simulink model "newController"  (R2023a)
settings: Solver=VariableStepAuto  StartTime=0.0  StopTime=10.0  RelTol=1e-3
libraries: ros2lib x65
(part 1 of 2)
settings Model: Creator=john  LastModifiedBy=john

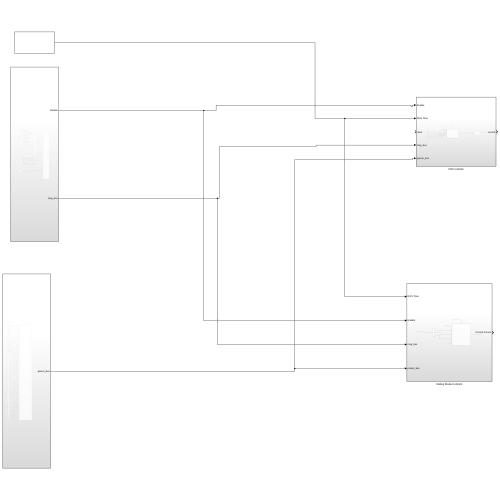
[thumbnail: Simulink's stored preview of the top-level diagram]
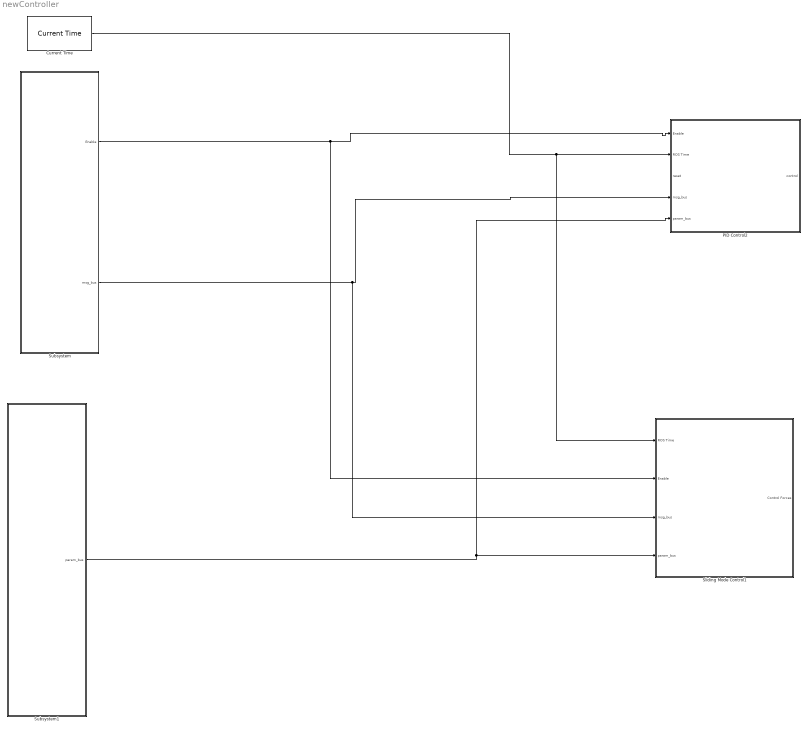
== system newController ==
  Current Time : ros2lib/Current Time  OutputFormat=bus  SampleTime=-1  ModelName=untitled
  PID Control2 : Subsystem
  Sliding Mode Control1 : Subsystem
  Subsystem : Subsystem
  Subsystem1 : Subsystem
  wires:
  Subsystem/2(msg_bus) -> Sliding Mode Control1/3(msg_bus), PID Control2/4(msg_bus)
  Subsystem1/1(param_bus) -> Sliding Mode Control1/4(param_bus), PID Control2/5(param_bus)
  Subsystem/1(Enable) -> Sliding Mode Control1/2(Enable), PID Control2/1(Enable)
  Current Time/1 -> Sliding Mode Control1/1(ROS Time), PID Control2/2(ROS Time)

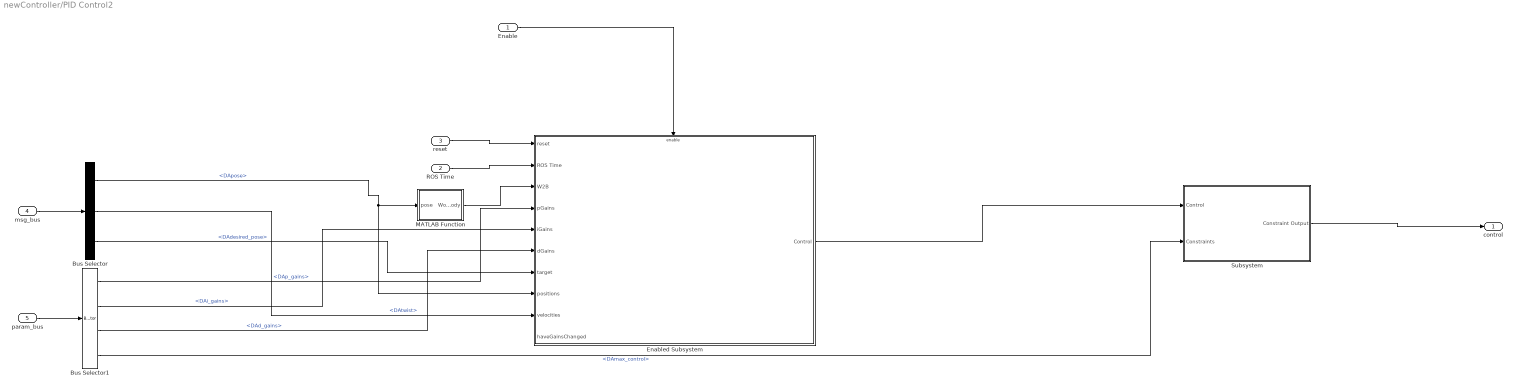
== system newController/PID Control2 ==
  Enable : Inport
  ROS Time : Inport  Port=2
  reset : Inport  Port=3
  msg_bus : Inport  Port=4
  param_bus : Inport  Port=5
  Bus Selector : BusSelector  OutputSignals=current_state.DApose,current_state.DAtwist,desired_pose.DAdesired_pose
  Bus Selector1 : BusSelector  OutputSignals=DAp_gains,DAi_gains,DAd_gains,DAmax_control
  Enabled Subsystem : Subsystem  TreatAsAtomicUnit=on
  MATLAB Function : MATLAB Function  TreatAsAtomicUnit=on
  Subsystem : Subsystem
  control : Outport
  wires:
  param_bus/1 -> Bus Selector1/1
  Enable/1 -> Enabled Subsystem/Enable
  reset/1 -> Enabled Subsystem/1(reset)
  ROS Time/1 -> Enabled Subsystem/2(ROS Time)
  Bus Selector1/1 -> Enabled Subsystem/4(pGains)  "<DAp_gains>"
  Bus Selector1/2 -> Enabled Subsystem/5(iGains)  "<DAi_gains>"
  Bus Selector1/3 -> Enabled Subsystem/6(dGains)  "<DAd_gains>"
  Bus Selector1/4 -> Subsystem/2(Constraints)  "<DAmax_control>"
  msg_bus/1 -> Bus Selector/1
  Bus Selector/1 -> MATLAB Function/1(pose), Enabled Subsystem/8(positions)  "<DApose>"
  Bus Selector/2 -> Enabled Subsystem/9(velocities)  "<DAtwist>"
  Bus Selector/3 -> Enabled Subsystem/7(target)  "<DAdesired_pose>"
  MATLAB Function/1(World2Body) -> Enabled Subsystem/3(W2B)
  Subsystem/1(Constraint Output) -> control/1
  Enabled Subsystem/1(Control) -> Subsystem/1(Control)

== system newController/Sliding Mode Control1 ==
  ROS Time : Inport
  Enable : Inport  Port=2
  msg_bus : Inport  Port=3
  param_bus : Inport  Port=4
  Bus Selector : BusSelector  OutputSignals=current_state.DApose,current_state.DAtwist,desired_pose.DAdesired_pose
  Subsystem : Subsystem
  Control Forces : Outport
  wires:
  msg_bus/1 -> Bus Selector/1
  ROS Time/1 -> Subsystem/1(ROS Time)
  Enable/1 -> Subsystem/Enable
  Bus Selector/1 -> Subsystem/2(Current Positions)  "<DApose>"
  Bus Selector/2 -> Subsystem/3(World Velocities)  "<DAtwist>"
  Bus Selector/3 -> Subsystem/4(Target Positions)  "<DAdesired_pose>"
  param_bus/1 -> Subsystem/5(param_bus)
  Subsystem/1(Control Forces) -> Control Forces/1

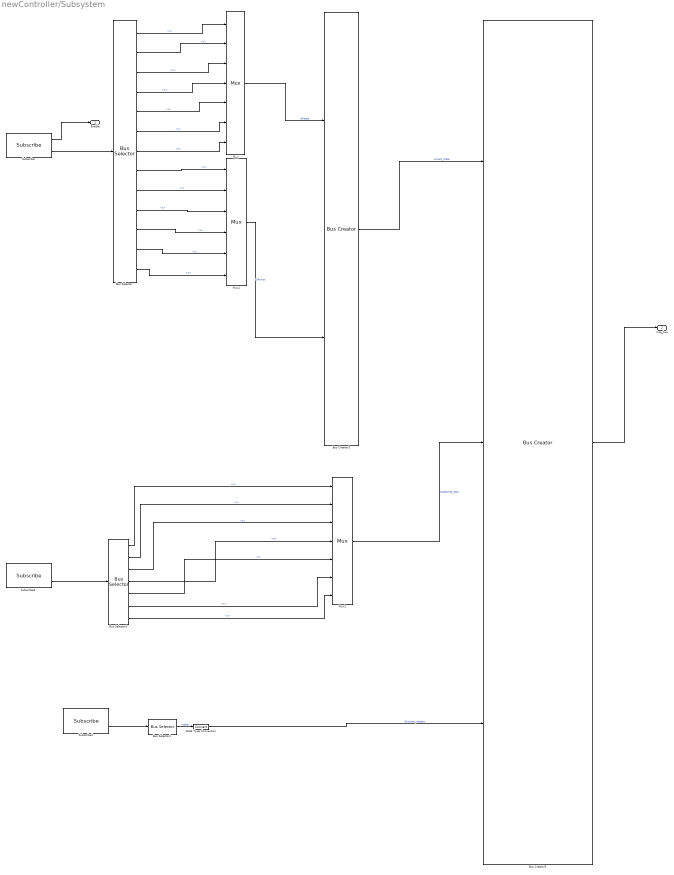
== system newController/Subsystem ==
  Bus Creator3 : BusCreator  Inputs=2
  Bus Creator5 : BusCreator  Inputs=3
  Bus Selector : BusSelector  OutputSignals=pose.pose.position.x,pose.pose.position.y,pose.pose.position.z,pose.pose.orientation.w,pose.pose.orientation.x,pose.pose.orientation.y,pose.pose.orientation.z,twist.twist.linear.x,twist.twist.linear.y,twist.twist.linear.z,twist.twist.angular.x,twist.twist.angular.y,twist.twist.angular.z
  Bus Selector1 : BusSelector  OutputSignals=data
  Bus Selector2 : BusSelector  OutputSignals=setpoint_vect.x,setpoint_vect.y,setpoint_vect.z,setpoint_quat.w,setpoint_quat.x,setpoint_quat.y,setpoint_quat.z
  Data Type Conversion : DataTypeConversion  SaturateOnIntegerOverflow=off  RndMeth=Floor
  Mux : Mux  Inputs=7
  Mux1 : Mux  Inputs=6
  Mux2 : Mux  Inputs=7
  Subscribe : ros2lib/Subscribe  topicSource=Specify your own  topic=/mercury/odometry/filtered  messageType=nav_msgs/Odometry  sampleTime=-1  QOSHistory=Keep last  QOSDepth=1  QOSReliability=Reliable  QOSDurability=Volatile
  Subscribe1 : ros2lib/Subscribe  topicSource=Specify your own  topic=/talos/controller/solver_weights  messageType=std_msgs/Int32MultiArray  sampleTime=-1  QOSHistory=Keep last  QOSDepth=1  QOSReliability=Reliable  QOSDurability=Volatile
      settings: LibrarySourceBlock=roslib/ROS 2/Subscribe
  Subscribe4 : ros2lib/Subscribe  topicSource=Specify your own  topic=/mercury/controller/desired  messageType=riptide_msgs2/ControllerCommand  sampleTime=-1  QOSHistory=Keep last  QOSDepth=1  QOSReliability=Reliable  QOSDurability=Volatile
  Enable : Outport
  msg_bus : Outport  Port=2
  wires:
  Subscribe/1 -> Enable/1
  Subscribe/2 -> Bus Selector/1
  Bus Selector/2 -> Mux/2  "<y>"
  Bus Selector/1 -> Mux/1  "<x>"
  Bus Selector/3 -> Mux/3  "<z>"
  Bus Selector/4 -> Mux/4  "<w>"
  Bus Selector/5 -> Mux/5  "<x>"
  Bus Selector/6 -> Mux/6  "<y>"
  Bus Selector/7 -> Mux/7  "<z>"
  Mux/1 -> Bus Creator3/1  "DApose"
  Bus Selector/8 -> Mux1/1  "<x>"
  Bus Selector/9 -> Mux1/2  "<y>"
  Bus Selector/10 -> Mux1/3  "<z>"
  Bus Selector/11 -> Mux1/4  "<x>"
  Bus Selector/12 -> Mux1/5  "<y>"
  Bus Selector/13 -> Mux1/6  "<z>"
  Mux1/1 -> Bus Creator3/2  "DAtwist"
  Subscribe4/2 -> Bus Selector2/1
  Bus Selector2/1 -> Mux2/1  "<x>"
  Bus Selector2/2 -> Mux2/2  "<y>"
  Bus Selector2/3 -> Mux2/3  "<z>"
  Bus Selector2/4 -> Mux2/4  "<w>"
  Bus Selector2/5 -> Mux2/5  "<x>"
  Bus Selector2/6 -> Mux2/6  "<y>"
  Bus Selector2/7 -> Mux2/7  "<z>"
  Bus Creator3/1 -> Bus Creator5/1  "current_state"
  Mux2/1 -> Bus Creator5/2  "DAdesired_pose"
  Bus Creator5/1 -> msg_bus/1
  Data Type Conversion/1 -> Bus Creator5/3  "DAsolver_weights"
  Subscribe1/2 -> Bus Selector1/1
  Bus Selector1/1 -> Data Type Conversion/1  "<data>"

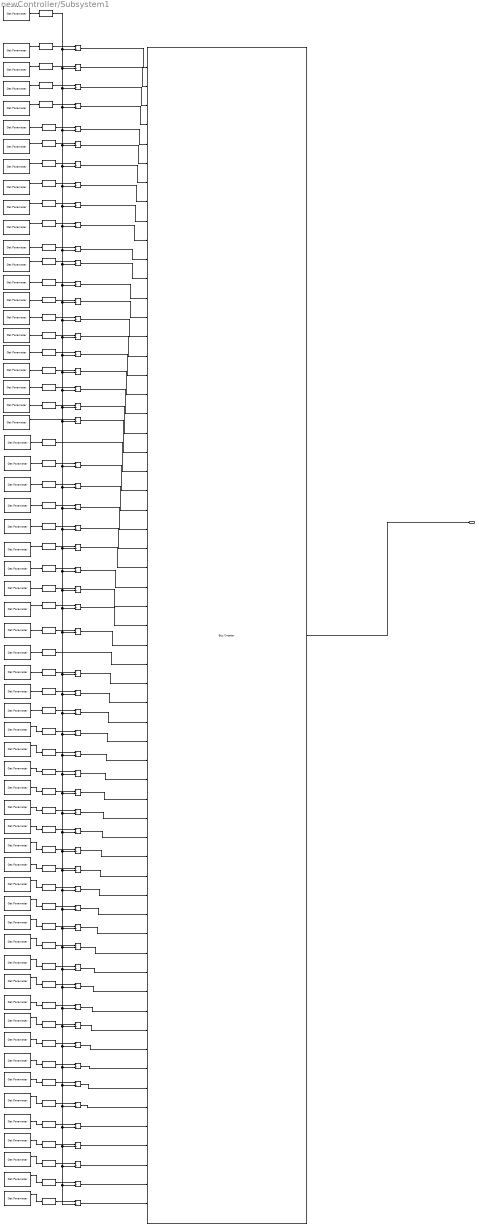
== system newController/Subsystem1 ==
  Active Input Mask : ros2lib/Get Parameter  ParameterName=controller__active_force_mask  ParameterType=int64[]  ParameterMaxArrayLength=6  ParameterInitialValue=[0,0,0,0,0,0]  SampleTime=-1  ModelName=mercury  BlockId=ParamGet_mercury_181
  Bsnt_safe_mode : DataTypeConversion  OutDataTypeStr=boolean  SaturateOnIntegerOverflow=off  RndMeth=Floor
  Bts_table_mode : DataTypeConversion  OutDataTypeStr=boolean  SaturateOnIntegerOverflow=off  RndMeth=Floor
  DAauto_tune_initial : Product  Inputs=*/
  DAauto_tune_mask : Product  Inputs=*/
  DAd_gains : Product  Inputs=*/
  DAi_gains : Product  Inputs=*/
  DAmax_control : Product  Inputs=*/
  DAnominal_variance : Product  Inputs=*/
  DAp_gains : Product  Inputs=*/
  DAsmc_eta_0 : Product  Inputs=*/
  DAsmc_eta_1 : Product  Inputs=*/
  DAsmc_lamda : Product  Inputs=*/
  DAsmc_max_accelerations : Product  Inputs=*/
  DAsmc_velocity_curve : Product  Inputs=*/
  DAtele_nudge_forces : Product  Inputs=*/
  DAts_rpm_coefficients : Product  Inputs=*/
  DAts_wrenchmat : Product  Inputs=*/
  Data Type Conversion{1,4..14,16..18,20..23} (19 alike) : DataTypeConversion  OutDataTypeStr=double  SaturateOnIntegerOverflow=off  RndMeth=Floor
  Dnominal_time{,1..17} (18 alike) : Product  Inputs=*/
  Dpositional_error_threshold : Product  Inputs=*/
  Dreset_threshold : Product  Inputs=*/
  Dreset_trust_threshold : Product  Inputs=*/
  Dreset_weight_minimum : Product  Inputs=*/
  Dsnt_barrel_roll_duration : Product  Inputs=*/
  Dsnt_barrel_roll_force : Product  Inputs=*/
  Dsnt_summersault_duration : Product  Inputs=*/
  Dsnt_summersault_force : Product  Inputs=*/
  Dtele_accel_force : Product  Inputs=*/
  Dtele_boost_cooldown : Product  Inputs=*/
  Dtele_boost_duration : Product  Inputs=*/
  Dtele_boost_multiplier : Product  Inputs=*/
  Dtele_drag_coefficient : Product  Inputs=*/
  Dtele_reverse_multiplier : Product  Inputs=*/
  Dtele_steering_angle : Product  Inputs=*/
  Dtele_throttle_deadzone : Product  Inputs=*/
  Dtele_width : Product  Inputs=*/
  Dtrust_decay_tau : Product  Inputs=*/
  Dtrust_growth_tau : Product  Inputs=*/
  Dts_disable_weight : Product  Inputs=*/
  Dts_feedback_decay : Product  Inputs=*/
  Dts_individual_thrust_limit : Product  Inputs=*/
  Dts_thrust_limit : Product  Inputs=*/
  Dvelocity_threshold : Product  Inputs=*/
  Eta 0 : ros2lib/Get Parameter  ParameterName=controller__SMC__SMC_params__eta_order_0  ParameterType=int64[]  ParameterMaxArrayLength=6  ParameterInitialValue=0.0  SampleTime=-1  ModelName=mercury  BlockId=ParamGet_mercury_260
      settings: LibrarySourceBlock=roslib/ROS 2/Get Parameter
  Eta 1 : ros2lib/Get Parameter  ParameterName=controller__SMC__SMC_params__eta_order_1  ParameterType=int64[]  ParameterMaxArrayLength=6  ParameterInitialValue=0.0  SampleTime=-1  ModelName=mercury  BlockId=ParamGet_mercury_261
      settings: LibrarySourceBlock=roslib/ROS 2/Get Parameter
  Force To Double{,1..38} (39 alike) : DataTypeConversion  OutDataTypeStr=double  SaturateOnIntegerOverflow=off  RndMeth=Floor
  Force To RPM Curve Parameters : ros2lib/Get Parameter  ParameterName=thruster_solver__force_to_rpm_coefficents  ParameterType=int64[]  ParameterMaxArrayLength=8  ParameterInitialValue=[0,0,0,0,0,0,0,0]  SampleTime=-1  ModelName=mercury  BlockId=ParamGet_mercury_301
      settings: LibrarySourceBlock=roslib/ROS 2/Get Parameter
  Get Parameter10 : ros2lib/Get Parameter  ParameterName=controller__pid__reset_threshold  ParameterType=int64  ParameterMaxArrayLength=16  ParameterInitialValue=100000  SampleTime=-1  ModelName=mercury  BlockId=ParamGet_mercury_302
      settings: LibrarySourceBlock=roslib/ROS 2/Get Parameter
  Get Parameter11 : ros2lib/Get Parameter  ParameterName=controller__teleop__width  ParameterType=int64  ParameterMaxArrayLength=16  ParameterInitialValue=900000  SampleTime=-1  ModelName=mercury  BlockId=ParamGet_mercury_303
  Get Parameter13 : ros2lib/Get Parameter  ParameterName=controller__stunt__summersault_duration  ParameterType=int64  ParameterMaxArrayLength=16  ParameterInitialValue=5000000.0  SampleTime=-1  ModelName=mercury  BlockId=ParamGet_mercury_304
  Get Parameter14 : ros2lib/Get Parameter  ParameterName=controller__stunt__summersault_force  ParameterType=int64  ParameterMaxArrayLength=16  ParameterInitialValue=20000000  SampleTime=-1  ModelName=mercury  BlockId=ParamGet_mercury_305
  Get Parameter15 : ros2lib/Get Parameter  ParameterName=controller__stunt__barrel_roll_duration  ParameterType=int64  ParameterMaxArrayLength=16  ParameterInitialValue=4000000.0  SampleTime=-1  ModelName=mercury  BlockId=ParamGet_mercury_306
  Get Parameter16 : ros2lib/Get Parameter  ParameterName=controller__teleop__boost__cooldown  ParameterType=int64  ParameterMaxArrayLength=16  ParameterInitialValue=10000000  SampleTime=-1  ModelName=mercury  BlockId=ParamGet_mercury_307
  Get Parameter17 : ros2lib/Get Parameter  ParameterName=controller__teleop__boost__duration  ParameterType=int64  ParameterMaxArrayLength=16  ParameterInitialValue=5000000  SampleTime=-1  ModelName=mercury  BlockId=ParamGet_mercury_308
  Get Parameter18 : ros2lib/Get Parameter  ParameterName=controller__teleop__boost__multiplier  ParameterType=int64  ParameterMaxArrayLength=16  ParameterInitialValue=1500000  SampleTime=-1  ModelName=mercury  BlockId=ParamGet_mercury_309
  Get Parameter19 : ros2lib/Get Parameter  ParameterName=controller__teleop__max_steering_angle  ParameterType=int64  ParameterMaxArrayLength=16  ParameterInitialValue=45000000  SampleTime=-1  ModelName=mercury  BlockId=ParamGet_mercury_310
  Get Parameter20 : ros2lib/Get Parameter  ParameterName=controller__teleop__nudge_forces  ParameterType=int64[]  ParameterMaxArrayLength=6  ParameterInitialValue=[20000000, 20000000, 2000000, 200000, 200000, 2000000]  SampleTime=-1  ModelName=mercury  BlockId=ParamGet_mercury_311
  Get Parameter21 : ros2lib/Get Parameter  ParameterName=controller__teleop__throttle_deadzone  ParameterType=int64  ParameterMaxArrayLength=16  ParameterInitialValue=50000  SampleTime=-1  ModelName=mercury  BlockId=ParamGet_mercury_312
  Get Parameter22 : ros2lib/Get Parameter  ParameterName=controller__teleop__reverse_force_multiplier  ParameterType=int64  ParameterMaxArrayLength=16  ParameterInitialValue=400000  SampleTime=-1  ModelName=mercury  BlockId=ParamGet_mercury_313
  Get Parameter23 : ros2lib/Get Parameter  ParameterName=controller__teleop__drag_coefficient  ParameterType=int64  ParameterMaxArrayLength=16  ParameterInitialValue=420000000  SampleTime=-1  ModelName=mercury  BlockId=ParamGet_mercury_314
  Get Parameter24 : ros2lib/Get Parameter  ParameterName=controller__teleop__accel_force  ParameterType=int64  ParameterMaxArrayLength=16  ParameterInitialValue=20000000  SampleTime=-1  ModelName=mercury  BlockId=ParamGet_mercury_315
  Get Parameter25 : ros2lib/Get Parameter  ParameterName=controller__stunt__safe_mode  ParameterType=boolean  ParameterMaxArrayLength=16  ParameterInitialValue=0  SampleTime=-1  ModelName=mercury  BlockId=ParamGet_mercury_316
  Get Parameter26 : ros2lib/Get Parameter  ParameterName=controller__stunt__barrel_roll_force  ParameterType=int64  ParameterMaxArrayLength=16  ParameterInitialValue=25000000.0  SampleTime=-1  ModelName=mercury  BlockId=ParamGet_mercury_317
  Get Thruster Wrench Matrix : ros2lib/Get Parameter  ParameterName=talos_wrenchmat  ParameterType=int64[]  ParameterMaxArrayLength=48  ParameterInitialValue=0.0  SampleTime=-1  ModelName=mercury  BlockId=ParamGet_mercury_318
      settings: LibrarySourceBlock=roslib/ROS 2/Get Parameter
  Iactive_input_mask : Product  Inputs=*/
  Individual Limit : ros2lib/Get Parameter  ParameterName=thruster_solver__individual_thrust_limit  ParameterType=int64  ParameterMaxArrayLength=16  ParameterInitialValue=5.0  SampleTime=-1  ModelName=mercury  BlockId=ParamGet_mercury_320
      settings: LibrarySourceBlock=roslib/ROS 2/Get Parameter
  Individual Limit1 : ros2lib/Get Parameter  ParameterName=thruster_solver__disable_weight  ParameterType=int64  ParameterMaxArrayLength=16  ParameterInitialValue=10000000  SampleTime=-1  ModelName=mercury  BlockId=ParamGet_mercury_321
      settings: LibrarySourceBlock=roslib/ROS 2/Get Parameter
  Individual Limit2 : ros2lib/Get Parameter  ParameterName=thruster_solver_table_mode  ParameterType=boolean  ParameterMaxArrayLength=16  ParameterInitialValue=false  SampleTime=-1  ModelName=mercury  BlockId=ParamGet_mercury_322
      settings: LibrarySourceBlock=roslib/ROS 2/Get Parameter
  Individual Limit3 : ros2lib/Get Parameter  ParameterName=thruster_solver__feedback_decay  ParameterType=int64  ParameterMaxArrayLength=16  ParameterInitialValue=1250000  SampleTime=-1  ModelName=mercury  BlockId=ParamGet_mercury_323
      settings: LibrarySourceBlock=roslib/ROS 2/Get Parameter
  Param Bus : BusCreator  Inputs=60
  Scaling Factor : ros2lib/Get Parameter  ParameterName=controller__SMC__SMC_params__scaling_factor  ParameterType=int64  ParameterMaxArrayLength=16  ParameterInitialValue=1000000  SampleTime=-1  ModelName=mercury  BlockId=ParamGet_mercury_325
      settings: LibrarySourceBlock=roslib/ROS 2/Get Parameter
  System Limit : ros2lib/Get Parameter  ParameterName=thruster_solver__system_thrust_limit  ParameterType=int64  ParameterMaxArrayLength=16  ParameterInitialValue=10  SampleTime=-1  ModelName=mercury  BlockId=ParamGet_mercury_326
      settings: LibrarySourceBlock=roslib/ROS 2/Get Parameter
  convergence threshold1 : ros2lib/Get Parameter  ParameterName=controller__feed_forward__auto_tune__auto_tune_mask  ParameterType=int64[]  ParameterMaxArrayLength=6  ParameterInitialValue=[0;0;0;0;0;0]  SampleTime=-1  ModelName=mercury  BlockId=ParamGet_mercury_327
      settings: LibrarySourceBlock=roslib/ROS 2/Get Parameter
  convergence threshold10 : ros2lib/Get Parameter  ParameterName=controller__feed_forward__auto_tune__trust_threshold  ParameterType=int64[]  ParameterMaxArrayLength=6  ParameterInitialValue=[970000, 970000, 970000, 970000, 970000, 970000]  SampleTime=-1  ModelName=mercury  BlockId=ParamGet_mercury_328
      settings: LibrarySourceBlock=roslib/ROS 2/Get Parameter
  convergence threshold11 : ros2lib/Get Parameter  ParameterName=controller__feed_forward__auto_tune__variation_threshold  ParameterType=int64[]  ParameterMaxArrayLength=6  ParameterInitialValue=[1000000, 1000000, 1000000, 1000000, 1000000, 1000000]  SampleTime=-1  ModelName=mercury  BlockId=ParamGet_mercury_329
      settings: LibrarySourceBlock=roslib/ROS 2/Get Parameter
  convergence threshold12 : ros2lib/Get Parameter  ParameterName=controller__feed_forward__auto_tune__axis_weights  ParameterType=int64[]  ParameterMaxArrayLength=6  ParameterInitialValue=[1000000, 1000000, 1000000, 1000000, 1000000, 1000000]  SampleTime=-1  ModelName=mercury  BlockId=ParamGet_mercury_330
      settings: LibrarySourceBlock=roslib/ROS 2/Get Parameter
  convergence threshold13 : ros2lib/Get Parameter  ParameterName=controller__feed_forward__auto_tune__variation_der_threshold  ParameterType=int64[]  ParameterMaxArrayLength=6  ParameterInitialValue=[1000000, 1000000, 1000000, 1000000, 1000000, 1000000]  SampleTime=-1  ModelName=mercury  BlockId=ParamGet_mercury_331
      settings: LibrarySourceBlock=roslib/ROS 2/Get Parameter
  convergence threshold14 : ros2lib/Get Parameter  ParameterName=inertia  ParameterType=int64[]  ParameterMaxArrayLength=3  ParameterInitialValue=[700000,1590000,1650000]  SampleTime=-1  ModelName=mercury  BlockId=ParamGet_mercury_332
      settings: LibrarySourceBlock=roslib/ROS 2/Get Parameter
  convergence threshold15 : ros2lib/Get Parameter  ParameterName=mass  ParameterType=int64  ParameterMaxArrayLength=6  ParameterInitialValue=32000000  SampleTime=-1  ModelName=mercury  BlockId=ParamGet_mercury_333
      settings: LibrarySourceBlock=roslib/ROS 2/Get Parameter
  convergence threshold16 : ros2lib/Get Parameter  ParameterName=controller__drag_compensator__apply_mask  ParameterType=int64[]  ParameterMaxArrayLength=36  ParameterInitialValue=zeros(36,1)  SampleTime=-1  ModelName=mercury  BlockId=ParamGet_mercury_334
      settings: LibrarySourceBlock=roslib/ROS 2/Get Parameter
  convergence threshold17 : ros2lib/Get Parameter  ParameterName=controller__drag_compensator__minimum_samples  ParameterType=int64  ParameterMaxArrayLength=6  ParameterInitialValue=60000000  SampleTime=-1  ModelName=mercury  BlockId=ParamGet_mercury_335
      settings: LibrarySourceBlock=roslib/ROS 2/Get Parameter
  convergence threshold18 : ros2lib/Get Parameter  ParameterName=controller__drag_compensator__minimum_absolute_velocity  ParameterType=int64  ParameterMaxArrayLength=6  ParameterInitialValue=200000  SampleTime=-1  ModelName=mercury  BlockId=ParamGet_mercury_336
      settings: LibrarySourceBlock=roslib/ROS 2/Get Parameter
  convergence threshold19 : ros2lib/Get Parameter  ParameterName=controller__drag_compensator__minimum_absolute_positional_error  ParameterType=int64  ParameterMaxArrayLength=3  ParameterInitialValue=200000  SampleTime=-1  ModelName=mercury  BlockId=ParamGet_mercury_337
      settings: LibrarySourceBlock=roslib/ROS 2/Get Parameter
  convergence threshold2 : ros2lib/Get Parameter  ParameterName=auto_ff__auto_ff  ParameterType=int64[]  ParameterMaxArrayLength=6  ParameterInitialValue=[0;0;0;0;0;0]  SampleTime=-1  ModelName=mercury  BlockId=ParamGet_mercury_338
      settings: LibrarySourceBlock=roslib/ROS 2/Get Parameter
  convergence threshold20 : ros2lib/Get Parameter  ParameterName=controller__drag_compensator__minimum_average_sampled_velocity  ParameterType=int64[]  ParameterMaxArrayLength=6  ParameterInitialValue=[100000,100000,100000,100000,100000,100000]  SampleTime=-1  ModelName=mercury  BlockId=ParamGet_mercury_339
      settings: LibrarySourceBlock=roslib/ROS 2/Get Parameter
  convergence threshold21 : ros2lib/Get Parameter  ParameterName=controller__drag_compensator__minimum_R2_coeffiecent  ParameterType=int64  ParameterMaxArrayLength=6  ParameterInitialValue=700000  SampleTime=-1  ModelName=mercury  BlockId=ParamGet_mercury_340
      settings: LibrarySourceBlock=roslib/ROS 2/Get Parameter
  convergence threshold22 : ros2lib/Get Parameter  ParameterName=controller__drag_compensator__learning_rate  ParameterType=int64  ParameterMaxArrayLength=6  ParameterInitialValue=200000  SampleTime=-1  ModelName=mercury  BlockId=ParamGet_mercury_341
      settings: LibrarySourceBlock=roslib/ROS 2/Get Parameter
  convergence threshold23 : ros2lib/Get Parameter  ParameterName=controller__drag_compensator__initial_compensation__forward  ParameterType=int64[]  ParameterMaxArrayLength=36  ParameterInitialValue=zeros(36,1)  SampleTime=-1  ModelName=mercury  BlockId=ParamGet_mercury_342
      settings: LibrarySourceBlock=roslib/ROS 2/Get Parameter
  convergence threshold24 : ros2lib/Get Parameter  ParameterName=controller__autoff__initial_ff  ParameterType=int64[]  ParameterMaxArrayLength=6  ParameterInitialValue=[0,0,0,0,0,0,0]  SampleTime=-1  ModelName=mercury  BlockId=ParamGet_mercury_343
      settings: LibrarySourceBlock=roslib/ROS 2/Get Parameter
  convergence threshold25 : ros2lib/Get Parameter  ParameterName=controller__drag_compensator__initial_compensation__reverse  ParameterType=int64[]  ParameterMaxArrayLength=36  ParameterInitialValue=zeros(36,1)  SampleTime=-1  ModelName=mercury  BlockId=ParamGet_mercury_344
      settings: LibrarySourceBlock=roslib/ROS 2/Get Parameter
  convergence threshold3 : ros2lib/Get Parameter  ParameterName=controller__controller_scale__trust_decay_tau  ParameterType=int64  ParameterMaxArrayLength=6  ParameterInitialValue=1000000  SampleTime=-1  ModelName=mercury  BlockId=ParamGet_mercury_345
      settings: LibrarySourceBlock=roslib/ROS 2/Get Parameter
  convergence threshold4 : ros2lib/Get Parameter  ParameterName=controller__controller_scale__trust_growth_tau  ParameterType=int64  ParameterMaxArrayLength=6  ParameterInitialValue=1000000  SampleTime=-1  ModelName=mercury  BlockId=ParamGet_mercury_346
      settings: LibrarySourceBlock=roslib/ROS 2/Get Parameter
  convergence threshold5 : ros2lib/Get Parameter  ParameterName=controller__controller_scale__reset_trust_threshold  ParameterType=int64  ParameterMaxArrayLength=200000  ParameterInitialValue=200000  SampleTime=-1  ModelName=mercury  BlockId=ParamGet_mercury_347
      settings: LibrarySourceBlock=roslib/ROS 2/Get Parameter
  convergence threshold6 : ros2lib/Get Parameter  ParameterName=controller__controller_scale__reset_weight_minimum  ParameterType=int64  ParameterMaxArrayLength=6  ParameterInitialValue=3000000  SampleTime=-1  ModelName=mercury  BlockId=ParamGet_mercury_348
      settings: LibrarySourceBlock=roslib/ROS 2/Get Parameter
  convergence threshold7 : ros2lib/Get Parameter  ParameterName=controller__controller_scale__nominal_variance  ParameterType=int64[]  ParameterMaxArrayLength=6  ParameterInitialValue=[0;0;0;0;0;0]  SampleTime=-1  ModelName=mercury  BlockId=ParamGet_mercury_349
      settings: LibrarySourceBlock=roslib/ROS 2/Get Parameter
  convergence threshold8 : ros2lib/Get Parameter  ParameterName=controller__controller_scale__nominal_time  ParameterType=int64  ParameterMaxArrayLength=6  ParameterInitialValue=3000000  SampleTime=-1  ModelName=mercury  BlockId=ParamGet_mercury_350
      settings: LibrarySourceBlock=roslib/ROS 2/Get Parameter
  convergence threshold9 : ros2lib/Get Parameter  ParameterName=controller__feed_forward__auto_tune__decay_factor  ParameterType=int64[]  ParameterMaxArrayLength=6  ParameterInitialValue=[200000, 200000, 200000, 200000, 200000, 200000]  SampleTime=-1  ModelName=mercury  BlockId=ParamGet_mercury_351
      settings: LibrarySourceBlock=roslib/ROS 2/Get Parameter
  d Gains : ros2lib/Get Parameter  ParameterName=controller__PID__d_gains  ParameterType=int64[]  ParameterMaxArrayLength=6  ParameterInitialValue=[0,0,0,0,0,0]  SampleTime=-1  ModelName=mercury  BlockId=ParamGet_mercury_352
      settings: LibrarySourceBlock=roslib/ROS 2/Get Parameter
  error threshold : ros2lib/Get Parameter  ParameterName=controller__feed_forward__auto_tune__positional_error_threshold  ParameterType=int64  ParameterMaxArrayLength=16  ParameterInitialValue=100000  SampleTime=-1  ModelName=mercury  BlockId=ParamGet_mercury_353
      settings: LibrarySourceBlock=roslib/ROS 2/Get Parameter
  i Gains : ros2lib/Get Parameter  ParameterName=controller__PID__i_gains  ParameterType=int64[]  ParameterMaxArrayLength=6  ParameterInitialValue=[0,0,0,0,0,0]  SampleTime=-1  ModelName=mercury  BlockId=ParamGet_mercury_354
      settings: LibrarySourceBlock=roslib/ROS 2/Get Parameter
  mass1 : ros2lib/Get Parameter  ParameterName=controller__SMC__SMC_params__velocity_curve_params  ParameterType=int64[]  ParameterMaxArrayLength=12  ParameterInitialValue=[0,0,0,0,0,0,0,0,0,0,0,0]  SampleTime=-1  ModelName=mercury  BlockId=ParamGet_mercury_355
      settings: LibrarySourceBlock=roslib/ROS 2/Get Parameter
  mass2 : ros2lib/Get Parameter  ParameterName=controller__SMC__max_target_accelerations  ParameterType=int64[]  ParameterMaxArrayLength=6  ParameterInitialValue=[10000,10000,10000,10000,10000,10000]  SampleTime=-1  ModelName=mercury  BlockId=ParamGet_mercury_356
      settings: LibrarySourceBlock=roslib/ROS 2/Get Parameter
  mass5 : ros2lib/Get Parameter  ParameterName=controller__SMC__SMC_params__lambda  ParameterType=int64[]  ParameterMaxArrayLength=6  ParameterInitialValue=0.0  SampleTime=-1  ModelName=mercury  BlockId=ParamGet_mercury_357
      settings: LibrarySourceBlock=roslib/ROS 2/Get Parameter
  max_control : ros2lib/Get Parameter  ParameterName=controller__PID__max_control_thresholds  ParameterType=int64[]  ParameterMaxArrayLength=6  ParameterInitialValue=[0,0,0,0,0,0]  SampleTime=-1  ModelName=mercury  BlockId=ParamGet_mercury_358
      settings: LibrarySourceBlock=roslib/ROS 2/Get Parameter
  p Gains : ros2lib/Get Parameter  ParameterName=controller__PID__p_gains  ParameterType=int64[]  ParameterMaxArrayLength=6  ParameterInitialValue=[0,0,0,0,0,0]  SampleTime=-1  ModelName=mercury  BlockId=ParamGet_mercury_359
      settings: LibrarySourceBlock=roslib/ROS 2/Get Parameter
  velocity threshold : ros2lib/Get Parameter  ParameterName=controller__feed_forward__auto_tune__velocity_threshold  ParameterType=int64  ParameterMaxArrayLength=16  ParameterInitialValue=100000  SampleTime=-1  ModelName=mercury  BlockId=ParamGet_mercury_360
      settings: LibrarySourceBlock=roslib/ROS 2/Get Parameter
  param_bus : Outport
  wires:
  Force To Double33/1 -> Dnominal_time10/1
  Data Type Conversion22/1 -> Dtele_boost_cooldown/1
  Force To Double30/1 -> Dnominal_time4/1
  Dsnt_barrel_roll_force/1 -> Param Bus/25  "Dsnt_barrel_roll_force"
  mass2/1 -> Data Type Conversion23/1
  p Gains/1 -> Force To Double6/1
  convergence threshold22/1 -> Force To Double35/1
  Dnominal_time13/1 -> Param Bus/55  "DAminimum_drag_update_velocity"
  Dnominal_time10/1 -> Param Bus/52  "Iminimum_drag_samples"
  Data Type Conversion7/1 -> DAsmc_eta_1/1
  Dnominal_time7/1 -> Param Bus/50  "Dmass"
  Force To Double26/1 -> Dnominal_time/1
  Eta 1/1 -> Data Type Conversion7/1
  Force To Double37/1 -> Dnominal_time16/1
  Force To Double20/1 -> DAauto_tune_initial/1
  Force To Double34/1 -> Dnominal_time8/1
  convergence threshold24/1 -> Force To Double37/1
  Data Type Conversion17/1 -> Dsnt_summersault_duration/1
  Dsnt_summersault_duration/1 -> Param Bus/24  "Dsnt_summersault_duration"
  convergence threshold17/1 -> Force To Double33/1
  Data Type Conversion16/1 -> Dsnt_summersault_force/1
  Dreset_threshold/1 -> Param Bus/5  "Dreset_threshold"
  Force To Double14/1 -> Dnominal_time5/1
  DAp_gains/1 -> Param Bus/2  "DAp_gains"
  System Limit/1 -> Force To Double1/1
  Dnominal_time2/1 -> Param Bus/45  "DAautoff_measurement_trust_threshold"
  Dnominal_time8/1 -> Param Bus/56  "Ddrag_minimum_correspondence_coeffiecent"
  Force To Double35/1 -> Dnominal_time14/1
  Force To Double9/1 -> Dreset_threshold/1
  Dtele_throttle_deadzone/1 -> Param Bus/11  "Dtele_throttle_deadzone"
  DAsmc_lamda/1 -> Param Bus/6  "DAsmc_lamda"
  convergence threshold23/1 -> Force To Double36/1
  Data Type Conversion5/1 -> DAsmc_lamda/1
  Dnominal_time9/1 -> Param Bus/51  "IAdrag_apply_mask"
  convergence threshold7/1 -> Force To Double25/1
  Data Type Conversion20/1 -> Dtele_boost_multiplier/1
  Dtele_steering_angle/1 -> Param Bus/13  "Dtele_steering_angle"
  Get Parameter22/1 -> Data Type Conversion13/1
  Dnominal_time14/1 -> Param Bus/57  "Ddrag_learning_rate"
  Get Parameter19/1 -> Data Type Conversion9/1
  DAtele_nudge_forces/1 -> Param Bus/12  "DAtele_nudge_forces"
  Dtele_reverse_multiplier/1 -> Param Bus/17  "Dtele_reverse_multiplier"
  Dnominal_time16/1 -> Param Bus/59  "DAautoff_init_compensation"
  Dreset_weight_minimum/1 -> Param Bus/41  "Dreset_weight_minimum"
  Force To Double1/1 -> Dts_thrust_limit/1
  Get Parameter25/1 -> Bsnt_safe_mode/1
  DAsmc_max_accelerations/1 -> Param Bus/10  "DAsmc_max_accelerations"
  Force To Double17/1 -> Dnominal_time11/1
  Data Type Conversion18/1 -> Dsnt_barrel_roll_force/1
  convergence threshold10/1 -> Force To Double28/1
  Get Parameter11/1 -> Data Type Conversion10/1
  convergence threshold16/1 -> Force To Double32/1
  Get Parameter16/1 -> Data Type Conversion22/1
  convergence threshold6/1 -> Force To Double24/1
  convergence threshold3/1 -> Force To Double21/1
  DAts_rpm_coefficients/1 -> Param Bus/30  "DAts_rpm_coefficients"
  Force To Double38/1 -> Dnominal_time17/1
  Dtele_boost_cooldown/1 -> Param Bus/20  "Dtele_boost_cooldown"
  Data Type Conversion6/1 -> DAsmc_eta_0/1
  Force To Double2/1 -> Dts_individual_thrust_limit/1
  Force To Double21/1 -> Dtrust_decay_tau/1
  Data Type Conversion11/1 -> Dtele_accel_force/1
  DAts_wrenchmat/1 -> Param Bus/27  "DAts_wrenchmat"
  convergence threshold2/1 -> Force To Double20/1
  Force To Double5/1 -> Dts_disable_weight/1
  Force To Double3/1 -> Dtele_throttle_deadzone/2, DAtele_nudge_forces/2, Dtele_steering_angle/2, Dtele_width/2, Dtele_accel_force/2, Dtele_drag_coefficient/2, Dtele_boost_multiplier/2, Dtele_boost_duration/2, Dtele_boost_cooldown/2, Dsnt_summersault_force/2, Dsnt_summersault_duration/2, Dsnt_barrel_roll_duration/2, DAts_wrenchmat/2, Dts_thrust_limit/2, Dts_individual_thrust_limit/2, DAts_rpm_coefficients/2, Dvelocity_threshold/2, Dtrust_decay_tau/2, Dtrust_growth_tau/2, Dreset_trust_threshold/2, Dreset_weight_minimum/2, DAnominal_variance/2, Dnominal_time17/2, Dnominal_time16/2, Dnominal_time15/2, Dnominal_time14/2, Dnominal_time8/2, Dnominal_time13/2, Dnominal_time12/2, Dnominal_time11/2, Dnominal_time10/2, Dnominal_time9/2, Dnominal_time7/2, Dnominal_time6/2, Dnominal_time5/2, Dnominal_time4/2, Dnominal_time3/2, Dnominal_time2/2, Dnominal_time1/2, Dnominal_time/2, DAauto_tune_initial/2, DAauto_tune_mask/2, Dpositional_error_threshold/2, Dts_feedback_decay/2, Dts_disable_weight/2, Dsnt_barrel_roll_force/2, Iactive_input_mask/2, Dtele_reverse_multiplier/2, DAsmc_max_accelerations/2, DAsmc_velocity_curve/2, DAsmc_eta_1/2, DAsmc_eta_0/2, DAsmc_lamda/2, Dreset_threshold/2, DAi_gains/2, DAd_gains/2, DAp_gains/2, DAmax_control/2
  Data Type Conversion10/1 -> Dtele_width/1
  DAsmc_velocity_curve/1 -> Param Bus/9  "DAsmc_velocity_curve"
  Force To Double15/1 -> Dnominal_time7/1
  Dnominal_time/1 -> Param Bus/43  "Dnominal_time"
  Get Parameter20/1 -> Data Type Conversion8/1
  convergence threshold1/1 -> Force To Double19/1
  Individual Limit/1 -> Force To Double2/1
  Dtele_drag_coefficient/1 -> Param Bus/16  "Dtele_drag_coefficient"
  Get Parameter21/1 -> Data Type Conversion4/1
  Force To Double22/1 -> Dtrust_growth_tau/1
  Dts_thrust_limit/1 -> Param Bus/28  "Dts_thrust_limit"
  Bsnt_safe_mode/1 -> Param Bus/22  "Bsnt_safe_mode"
  i Gains/1 -> Force To Double8/1
  convergence threshold12/1 -> Force To Double30/1
  Param Bus/1 -> param_bus/1
  Scaling Factor/1 -> Force To Double3/1
  Force To Double10/1 -> Dts_feedback_decay/1
  Data Type Conversion21/1 -> Dtele_boost_duration/1
  Dtele_accel_force/1 -> Param Bus/15  "Dtele_accel_force"
  Data Type Conversion13/1 -> Dtele_reverse_multiplier/1
  Force To Double8/1 -> DAi_gains/1
  Dts_individual_thrust_limit/1 -> Param Bus/29  "Dts_individual_thrust_limit"
  convergence threshold11/1 -> Force To Double29/1
  Data Type Conversion1/1 -> DAsmc_velocity_curve/1
  Get Parameter18/1 -> Data Type Conversion20/1
  convergence threshold21/1 -> Force To Double34/1
  Dnominal_time11/1 -> Param Bus/53  "Dminimum_drag_sampling_velocity"
  convergence threshold9/1 -> Force To Double27/1
  convergence threshold8/1 -> Force To Double26/1
  Dnominal_time15/1 -> Param Bus/58  "DAdrag_init_compensation_forward"
  convergence threshold15/1 -> Force To Double15/1
  Force To RPM Curve Parameters/1 -> Force To Double4/1
  convergence threshold5/1 -> Force To Double23/1
  Dsnt_summersault_force/1 -> Param Bus/23  "Dsnt_summersault_force"
  Force To Double11/1 -> DAmax_control/1
  Get Parameter10/1 -> Force To Double9/1
  mass1/1 -> Data Type Conversion1/1
  Dnominal_time1/1 -> Param Bus/44  "DAautoff_body_force_decay_percentage"
  DAauto_tune_mask/1 -> Param Bus/36  "DAauto_tune_mask"
  Data Type Conversion23/1 -> DAsmc_max_accelerations/1
  max_control/1 -> Force To Double11/1
  Dnominal_time3/1 -> Param Bus/46  "DAautoff_standard_variation_threshold"
  Bts_table_mode/1 -> Param Bus/32  "Bts_table_mode"
  Force To Double29/1 -> Dnominal_time3/1
  Dtele_boost_duration/1 -> Param Bus/19  "Dtele_boost_duration"
  Iactive_input_mask/1 -> Param Bus/21  "Iactive_input_mask"
  Get Thruster Wrench Matrix/1 -> Force To Double/1
  convergence threshold4/1 -> Force To Double22/1
  Data Type Conversion9/1 -> Dtele_steering_angle/1
  Data Type Conversion4/1 -> Dtele_throttle_deadzone/1
  d Gains/1 -> Force To Double7/1
  Force To Double24/1 -> Dreset_weight_minimum/1
  DAsmc_eta_1/1 -> Param Bus/8  "DAsmc_eta_1"
  Force To Double7/1 -> DAd_gains/1
  Individual Limit2/1 -> Bts_table_mode/1
  Data Type Conversion8/1 -> DAtele_nudge_forces/1
  Force To Double23/1 -> Dreset_trust_threshold/1
  Force To Double6/1 -> DAp_gains/1
  Get Parameter13/1 -> Data Type Conversion17/1
  Data Type Conversion12/1 -> Dtele_drag_coefficient/1
  Dnominal_time4/1 -> Param Bus/47  "DAautoff_active_force_weights"
  Dts_disable_weight/1 -> Param Bus/31  "Dts_disable_weight"
  Get Parameter24/1 -> Data Type Conversion11/1
  DAd_gains/1 -> Param Bus/3  "DAd_gains"
  Dtrust_decay_tau/1 -> Param Bus/38  "Dtrust_decay_tau"
  Force To Double4/1 -> DAts_rpm_coefficients/1
  DAmax_control/1 -> Param Bus/1  "DAmax_control"
  Dpositional_error_threshold/1 -> Param Bus/34  "Dpositional_error_threshold"
  Get Parameter14/1 -> Data Type Conversion16/1
  Force To Double16/1 -> Dnominal_time6/1
  Dvelocity_threshold/1 -> Param Bus/35  "Dvelocity_threshold"
  velocity threshold/1 -> Force To Double13/1
  Dtele_boost_multiplier/1 -> Param Bus/18  "Dtele_boost_multiplier"
  convergence threshold18/1 -> Force To Double17/1
  Force To Double12/1 -> Dpositional_error_threshold/1
  Force To Double/1 -> DAts_wrenchmat/1
  Data Type Conversion14/1 -> Dsnt_barrel_roll_duration/1
  DAauto_tune_initial/1 -> Param Bus/37  "DAauto_tune_initial"
  DAsmc_eta_0/1 -> Param Bus/7  "DAsmc_eta_0"
  Dreset_trust_threshold/1 -> Param Bus/40  "Dreset_trust_threshold"
  DAnominal_variance/1 -> Param Bus/42  "DAnominal_variance"
  Dtrust_growth_tau/1 -> Param Bus/39  "Dtrust_growth_tau"
  Dnominal_time12/1 -> Param Bus/54  "Dminimum_drag_positional_error"
  Force To Double27/1 -> Dnominal_time1/1
  Individual Limit3/1 -> Force To Double10/1
  Force To Double19/1 -> DAauto_tune_mask/1
  Force To Double36/1 -> Dnominal_time15/1
  Active Input Mask/1 -> Iactive_input_mask/1
  convergence threshold20/1 -> Force To Double18/1
  mass5/1 -> Data Type Conversion5/1
  Force To Double13/1 -> Dvelocity_threshold/1
  Force To Double31/1 -> Dnominal_time12/1
  Individual Limit1/1 -> Force To Double5/1
  Dts_feedback_decay/1 -> Param Bus/33  "Dts_feedback_decay"
  Dnominal_time5/1 -> Param Bus/48  "DAautoff_variation_derivative_threshold"
  Get Parameter23/1 -> Data Type Conversion12/1
  Eta 0/1 -> Data Type Conversion6/1
  Dtele_width/1 -> Param Bus/14  "Dtele_width"
  convergence threshold14/1 -> Force To Double16/1
  Dnominal_time6/1 -> Param Bus/49  "DAinterias"
  Get Parameter15/1 -> Data Type Conversion14/1
  convergence threshold19/1 -> Force To Double31/1
  DAi_gains/1 -> Param Bus/4  "DAi_gains"
  convergence threshold25/1 -> Force To Double38/1
  Get Parameter17/1 -> Data Type Conversion21/1
  Force To Double18/1 -> Dnominal_time13/1
  Force To Double25/1 -> DAnominal_variance/1
  Force To Double32/1 -> Dnominal_time9/1
  convergence threshold13/1 -> Force To Double14/1
  Dnominal_time17/1 -> Param Bus/60  "DAdrag_init_compensation_reverse"
  error threshold/1 -> Force To Double12/1
  Dsnt_barrel_roll_duration/1 -> Param Bus/26  "Dsnt_barrel_roll_duration"
  Force To Double28/1 -> Dnominal_time2/1
  Get Parameter26/1 -> Data Type Conversion18/1

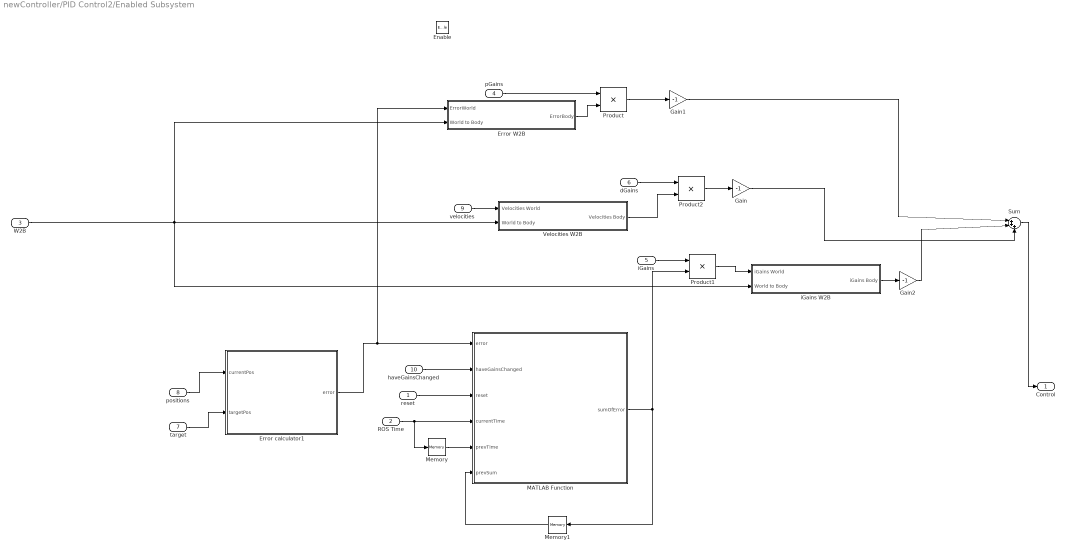
== system newController/PID Control2/Enabled Subsystem ==
  reset : Inport
  ROS Time : Inport  Port=2
  W2B : Inport  Port=3
  pGains : Inport  Port=4
  iGains : Inport  Port=5
  dGains : Inport  Port=6
  target : Inport  Port=7
  positions : Inport  Port=8
  velocities : Inport  Port=9
  haveGainsChanged : Inport  Port=10
  Enable : EnablePort
  Error W2B : Subsystem
  Error calculator1 : MATLAB Function  TreatAsAtomicUnit=on
  Gain : Gain  Gain=-1
  Gain1 : Gain  Gain=-1
  Gain2 : Gain  Gain=-1
  MATLAB Function : MATLAB Function  TreatAsAtomicUnit=on
  Memory : Memory  InheritSampleTime=on
  Memory1 : Memory  InheritSampleTime=on
  Product : Product
  Product1 : Product
  Product2 : Product
  Sum : Sum  Inputs=|+++
  Velocities W2B : Subsystem
  iGains W2B : Subsystem
  Control : Outport
  wires:
  positions/1 -> Error calculator1/1(currentPos)
  target/1 -> Error calculator1/2(targetPos)
  Error calculator1/1(error) -> MATLAB Function/1(error), Error W2B/1(ErrorWorld)
  reset/1 -> MATLAB Function/3(reset)
  ROS Time/1 -> Memory/1, MATLAB Function/4(currentTime)
  haveGainsChanged/1 -> MATLAB Function/2(haveGainsChanged)
  Memory/1 -> MATLAB Function/5(prevTime)
  MATLAB Function/1(sumOfError) -> Product1/2, Memory1/1
  Memory1/1 -> MATLAB Function/6(prevSum)
  iGains/1 -> Product1/1
  velocities/1 -> Velocities W2B/1(Velocities World)
  Product2/1 -> Gain/1
  Product/1 -> Gain1/1
  Gain/1 -> Sum/3
  Sum/1 -> Control/1
  dGains/1 -> Product2/1
  W2B/1 -> iGains W2B/2(World to Body), Velocities W2B/2(World to Body), Error W2B/2(World to Body)
  Error W2B/1(ErrorBody) -> Product/2
  pGains/1 -> Product/1
  iGains W2B/1(iGains Body) -> Gain2/1
  Product1/1 -> iGains W2B/1(iGains World)
  Velocities W2B/1(Velocities Body) -> Product2/2
  Gain1/1 -> Sum/1
  Gain2/1 -> Sum/2

== system newController/PID Control2/Subsystem ==
  Control : Inport
  Constraints : Inport  Port=2
  Gain : Gain  Gain=-1
  MinMax : MinMax  Function=max  Inputs=2
  MinMax1 : MinMax  Inputs=2
  Constraint Output : Outport
  wires:
  Constraints/1 -> MinMax1/2, Gain/1
  Gain/1 -> MinMax/2
  Control/1 -> MinMax/1
  MinMax/1 -> MinMax1/1
  MinMax1/1 -> Constraint Output/1

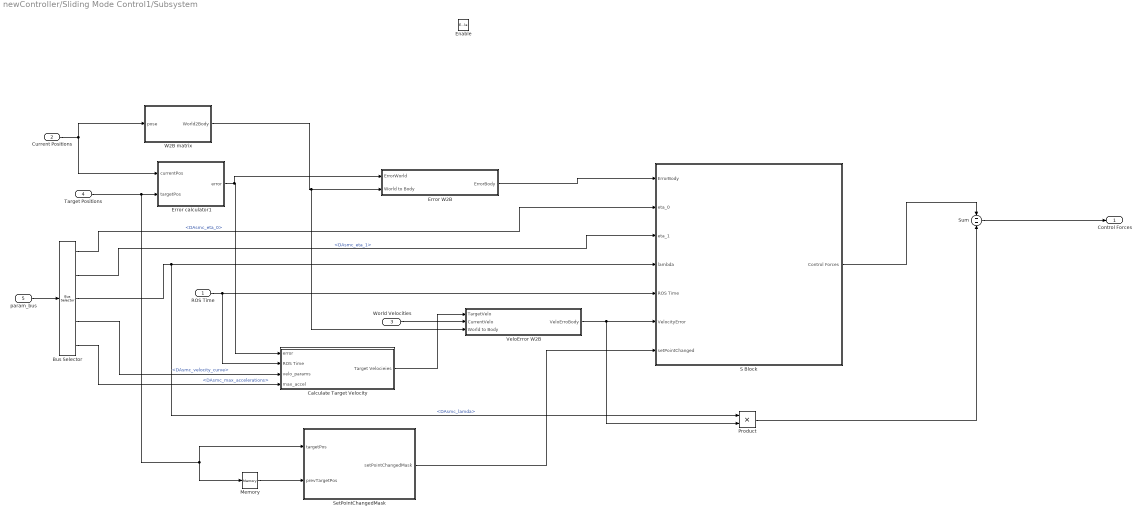
== system newController/Sliding Mode Control1/Subsystem ==
  ROS Time : Inport
  Current Positions : Inport  Port=2
  World Velocities : Inport  Port=3
  Target Positions : Inport  Port=4
  param_bus : Inport  Port=5
  Enable : EnablePort
  Bus Selector : BusSelector  OutputSignals=DAsmc_eta_0,DAsmc_eta_1,DAsmc_lamda,DAsmc_velocity_curve,DAsmc_max_accelerations
  Calculate Target Velocity : Subsystem
  Error W2B : Subsystem
  Error calculator1 : MATLAB Function  TreatAsAtomicUnit=on
  Memory : Memory
  Product : Product
  S Block : Subsystem
  SetPointChangedMask : MATLAB Function  TreatAsAtomicUnit=on
  Sum : Sum  Inputs=--
  VeloError W2B : Subsystem
  W2B matrix : MATLAB Function  TreatAsAtomicUnit=on
  Control Forces : Outport
  wires:
  Target Positions/1 -> Memory/1, SetPointChangedMask/1(targetPos), Error calculator1/2(targetPos)
  Current Positions/1 -> W2B matrix/1(pose), Error calculator1/1(currentPos)
  ROS Time/1 -> Calculate Target Velocity/2(ROS Time), S Block/5(ROS Time)
  Error calculator1/1(error) -> Error W2B/1(ErrorWorld), Calculate Target Velocity/1(error)
  param_bus/1 -> Bus Selector/1
  Bus Selector/5 -> Calculate Target Velocity/4(max_accel)  "<DAsmc_max_accelerations>"
  Bus Selector/4 -> Calculate Target Velocity/3(velo_params)  "<DAsmc_velocity_curve>"
  Bus Selector/2 -> S Block/3(eta_1)  "<DAsmc_eta_1>"
  Bus Selector/1 -> S Block/2(eta_0)  "<DAsmc_eta_0>"
  Bus Selector/3 -> S Block/4(lambda), Product/1  "<DAsmc_lamda>"
  World Velocities/1 -> VeloError W2B/2(CurrentVelo)
  Calculate Target Velocity/1(Target Velocieies) -> VeloError W2B/1(TargetVelo)
  Error W2B/1(ErrorBody) -> S Block/1(ErrorBody)
  W2B matrix/1(World2Body) -> VeloError W2B/3(World to Body), Error W2B/2(World to Body)
  VeloError W2B/1(VeloErroBody) -> Product/2, S Block/6(VelocityError)
  Memory/1 -> SetPointChangedMask/2(prevTargetPos)
  SetPointChangedMask/1(setPointChangedMask) -> S Block/7(setPointChanged)
  S Block/1(Control Forces) -> Sum/1
  Sum/1 -> Control Forces/1
  Product/1 -> Sum/2

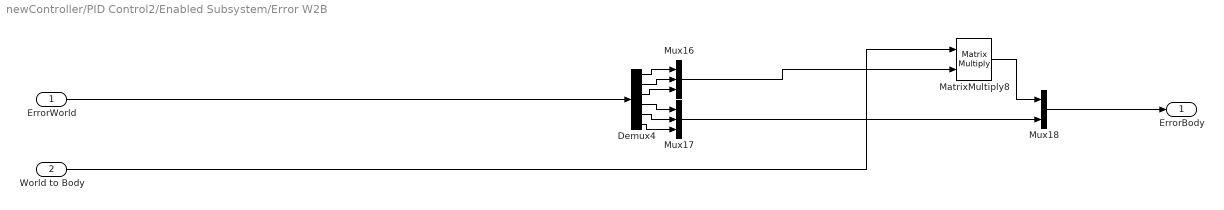
== system newController/PID Control2/Enabled Subsystem/Error W2B ==
  ErrorWorld : Inport
  World to Body : Inport  Port=2
  Demux4 : Demux  Outputs=6
  MatrixMultiply8 : Product  Multiplication=Matrix(*)
  Mux16 : Mux  Inputs=3
  Mux17 : Mux  Inputs=3
  Mux18 : Mux  Inputs=2
  ErrorBody : Outport
  wires:
  Demux4/2 -> Mux16/2
  Demux4/4 -> Mux17/1
  Mux16/1 -> MatrixMultiply8/2
  Demux4/6 -> Mux17/3
  Demux4/1 -> Mux16/1
  Demux4/5 -> Mux17/2
  Mux17/1 -> Mux18/2
  ErrorWorld/1 -> Demux4/1
  Demux4/3 -> Mux16/3
  MatrixMultiply8/1 -> Mux18/1
  Mux18/1 -> ErrorBody/1
  World to Body/1 -> MatrixMultiply8/1

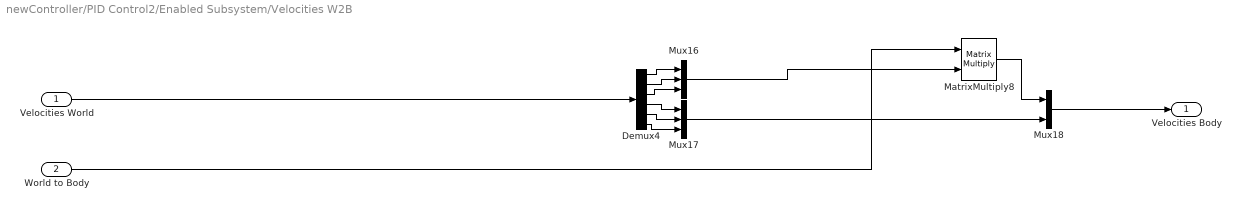
== system newController/PID Control2/Enabled Subsystem/Velocities W2B ==
  Velocities World : Inport
  World to Body : Inport  Port=2
  Demux4 : Demux  Outputs=6
  MatrixMultiply8 : Product  Multiplication=Matrix(*)
  Mux16 : Mux  Inputs=3
  Mux17 : Mux  Inputs=3
  Mux18 : Mux  Inputs=2
  Velocities Body : Outport
  wires:
  Demux4/2 -> Mux16/2
  Demux4/4 -> Mux17/1
  Mux16/1 -> MatrixMultiply8/2
  Demux4/6 -> Mux17/3
  Demux4/1 -> Mux16/1
  Demux4/5 -> Mux17/2
  Mux17/1 -> Mux18/2
  Velocities World/1 -> Demux4/1
  Demux4/3 -> Mux16/3
  MatrixMultiply8/1 -> Mux18/1
  Mux18/1 -> Velocities Body/1
  World to Body/1 -> MatrixMultiply8/1

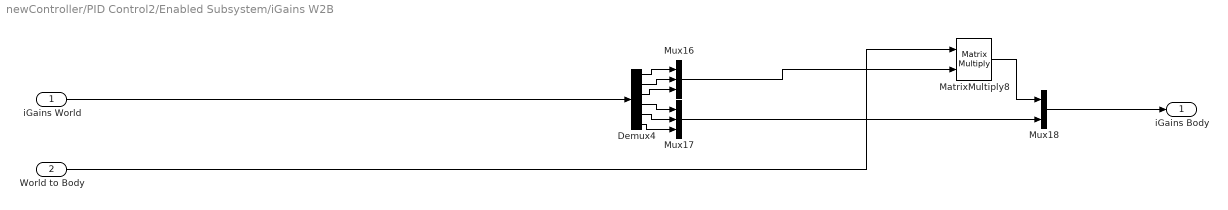
== system newController/PID Control2/Enabled Subsystem/iGains W2B ==
  iGains World : Inport
  World to Body : Inport  Port=2
  Demux4 : Demux  Outputs=6
  MatrixMultiply8 : Product  Multiplication=Matrix(*)
  Mux16 : Mux  Inputs=3
  Mux17 : Mux  Inputs=3
  Mux18 : Mux  Inputs=2
  iGains Body : Outport
  wires:
  Demux4/2 -> Mux16/2
  Demux4/4 -> Mux17/1
  Mux16/1 -> MatrixMultiply8/2
  Demux4/6 -> Mux17/3
  Demux4/1 -> Mux16/1
  Demux4/5 -> Mux17/2
  Mux17/1 -> Mux18/2
  iGains World/1 -> Demux4/1
  Demux4/3 -> Mux16/3
  MatrixMultiply8/1 -> Mux18/1
  Mux18/1 -> iGains Body/1
  World to Body/1 -> MatrixMultiply8/1

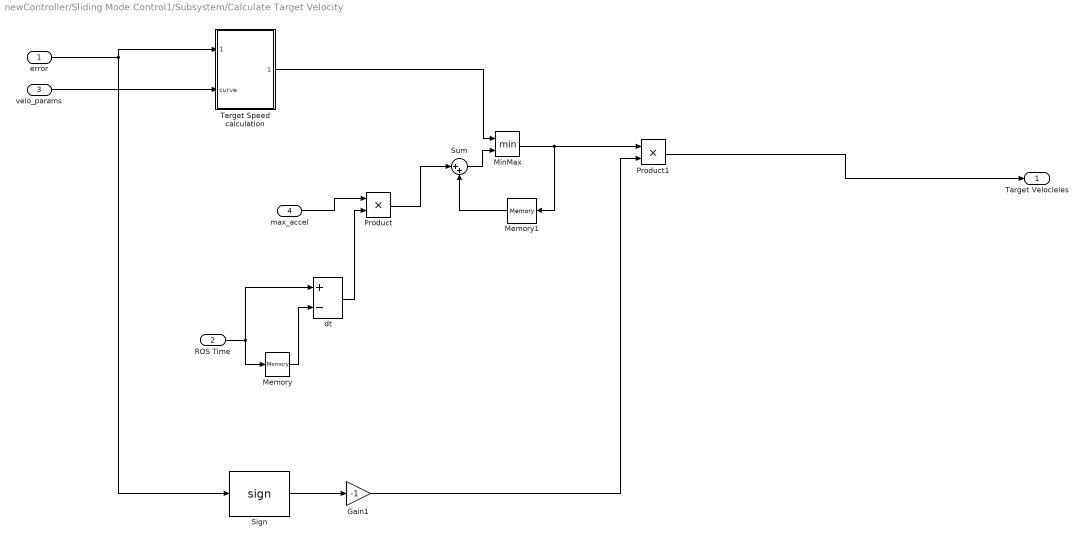
== system newController/Sliding Mode Control1/Subsystem/Calculate Target Velocity ==
  error : Inport
  ROS Time : Inport  Port=2
  velo_params : Inport  Port=3
  max_accel : Inport  Port=4
  Gain1 : Gain  Gain=-1
  Memory : Memory
  Memory1 : Memory
  MinMax : MinMax  Inputs=2
  Product : Product
  Product1 : Product
  Sign : Signum
  Sum : Sum  Inputs=|++
  Target Speed calculation : MATLAB Function  TreatAsAtomicUnit=on
  dt : Sum  Inputs=+-
  Target Velocieies : Outport
  wires:
  error/1 -> Sign/1, Target Speed calculation/1(posError)
  ROS Time/1 -> Memory/1, dt/1
  Memory/1 -> dt/2
  velo_params/1 -> Target Speed calculation/2(curve)
  Target Speed calculation/1(targetSpeed) -> MinMax/1
  max_accel/1 -> Product/1
  dt/1 -> Product/2
  Product/1 -> Sum/1
  MinMax/1 -> Product1/1, Memory1/1
  Memory1/1 -> Sum/2
  Sum/1 -> MinMax/2
  Sign/1 -> Gain1/1
  Product1/1 -> Target Velocieies/1
  Gain1/1 -> Product1/2

== system newController/Sliding Mode Control1/Subsystem/Error W2B ==
  ErrorWorld : Inport
  World to Body : Inport  Port=2
  Demux4 : Demux  Outputs=6
  MatrixMultiply8 : Product  Multiplication=Matrix(*)
  Mux16 : Mux  Inputs=3
  Mux17 : Mux  Inputs=3
  Mux18 : Mux  Inputs=2
  ErrorBody : Outport
  wires:
  Demux4/2 -> Mux16/2
  Demux4/4 -> Mux17/1
  Mux16/1 -> MatrixMultiply8/2
  Demux4/6 -> Mux17/3
  Demux4/1 -> Mux16/1
  Demux4/5 -> Mux17/2
  Mux17/1 -> Mux18/2
  ErrorWorld/1 -> Demux4/1
  Demux4/3 -> Mux16/3
  MatrixMultiply8/1 -> Mux18/1
  Mux18/1 -> ErrorBody/1
  World to Body/1 -> MatrixMultiply8/1

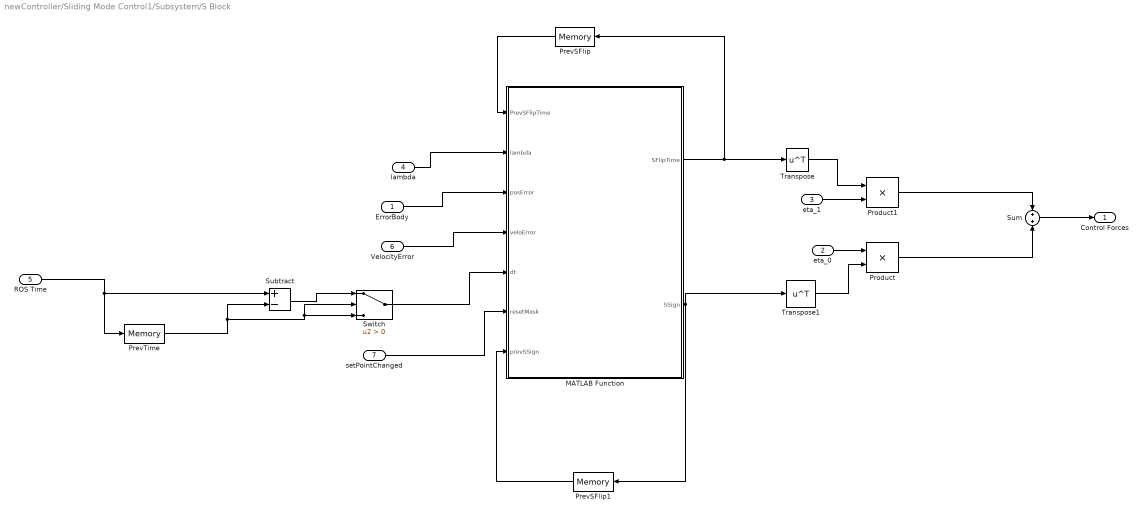
== system newController/Sliding Mode Control1/Subsystem/S Block ==
  ErrorBody : Inport
  eta_0 : Inport  Port=2
  eta_1 : Inport  Port=3
  lambda : Inport  Port=4
  ROS Time : Inport  Port=5
  VelocityError : Inport  Port=6
  setPointChanged : Inport  Port=7
  MATLAB Function : MATLAB Function  TreatAsAtomicUnit=on
  PrevSFlip : Memory  InitialCondition=[0;0;0;0;0;0]
  PrevSFlip1 : Memory  InitialCondition=[0;0;0;0;0;0]
  PrevTime : Memory
  Product : Product
  Product1 : Product
  Subtract : Sum  Inputs=+-
  Sum : Sum
  Switch : Switch  Criteria=u2 > Threshold  SaturateOnIntegerOverflow=off  InputSameDT=off
  Transpose : Math  Operator=transpose  OutputSignalType=real
  Transpose1 : Math  Operator=transpose  OutputSignalType=real
  Control Forces : Outport
  wires:
  eta_0/1 -> Product/1
  MATLAB Function/2(SSign) -> PrevSFlip1/1, Transpose1/1
  eta_1/1 -> Product1/2
  MATLAB Function/1(SFlipTime) -> Transpose/1, PrevSFlip/1
  Product/1 -> Sum/2
  Sum/1 -> Control Forces/1
  lambda/1 -> MATLAB Function/2(lambda)
  ErrorBody/1 -> MATLAB Function/3(posError)
  VelocityError/1 -> MATLAB Function/4(veloError)
  PrevSFlip/1 -> MATLAB Function/1(PrevSFlipTime)
  ROS Time/1 -> PrevTime/1, Subtract/1
  Subtract/1 -> Switch/1
  Switch/1 -> MATLAB Function/5(dt)
  PrevTime/1 -> Switch/3, Switch/2, Subtract/2
  setPointChanged/1 -> MATLAB Function/6(resetMask)
  Transpose/1 -> Product1/1
  PrevSFlip1/1 -> MATLAB Function/7(prevSSign)
  Transpose1/1 -> Product/2
  Product1/1 -> Sum/1

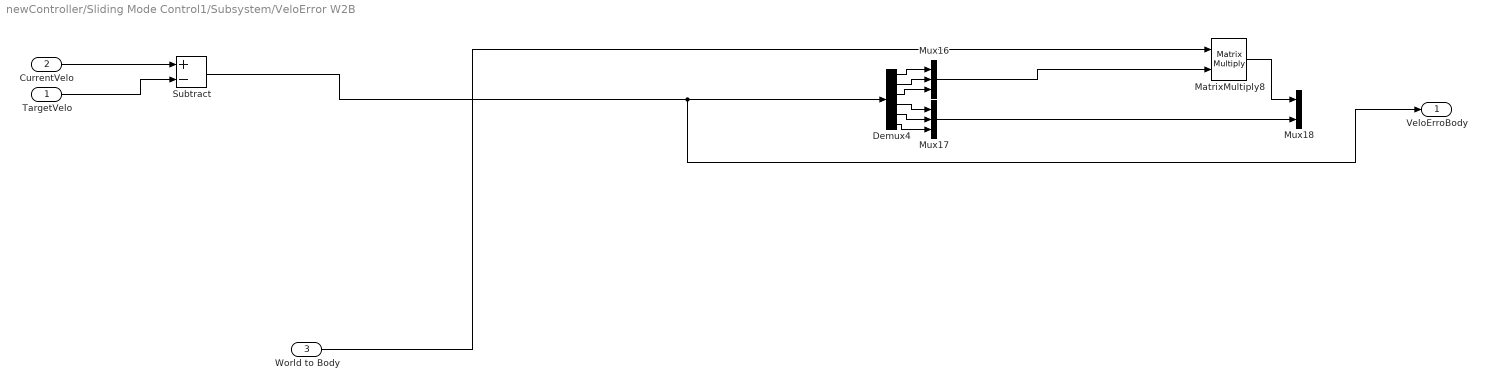
== system newController/Sliding Mode Control1/Subsystem/VeloError W2B ==
  TargetVelo : Inport
  CurrentVelo : Inport  Port=2
  World to Body : Inport  Port=3
  Demux4 : Demux  Outputs=6
  MatrixMultiply8 : Product  Multiplication=Matrix(*)
  Mux16 : Mux  Inputs=3
  Mux17 : Mux  Inputs=3
  Mux18 : Mux  Inputs=2
  Subtract : Sum  Inputs=+-
  VeloErroBody : Outport
  wires:
  Demux4/2 -> Mux16/2
  Demux4/4 -> Mux17/1
  Mux16/1 -> MatrixMultiply8/2
  Demux4/6 -> Mux17/3
  Demux4/1 -> Mux16/1
  Demux4/5 -> Mux17/2
  Mux17/1 -> Mux18/2
  TargetVelo/1 -> Subtract/2
  Demux4/3 -> Mux16/3
  MatrixMultiply8/1 -> Mux18/1
  World to Body/1 -> MatrixMultiply8/1
  CurrentVelo/1 -> Subtract/1
  Subtract/1 -> VeloErroBody/1, Demux4/1

== matlab function newController/PID Control2/Enabled Subsystem/Error calculator1 ==
  data: currentPos input; targetPos input; error output
function error = fcn(currentPos, targetPos)

error = zeros(1,6);

%World Frame linear error
eWorld = zeros(1,3);

eWorld(1) = targetPos(1) - currentPos(1);
eWorld(2) = targetPos(2) - currentPos(2);
eWorld(3) = targetPos(3) - currentPos(3);

%Quaternion that represents position
currentQuat = [currentPos(7), currentPos(4), currentPos(5), currentPos(6)];

%make it a unit quaternion
unitQuat = currentQuat ./ norm(currentQuat);

%quaternion that we want to be at
setQuat = [targetPos(7), -targetPos(4), -targetPos(5), -targetPos(6)];

uSetQuat = setQuat ./ norm(setQuat);

%multiply the inverse of the unit quat by the set quat to get an error
eQuat = quatmultiply(uSetQuat, conj(unitQuat));
if(eQuat(1) < 0) 
    eQuat = -eQuat;
end

%total rotation angle
w = max(min(eQuat(1),1),-1);
theta = 2 * acos(w);

%sin(theta/2)
s = sqrt(max(1 - w^2,0));

%rotation axis and rotation vector
if s < 1e-6
   eRot = [0 0 0];
else
   axis = eQuat(2:4) / s;
   eRot = theta * axis;
end

theta_mag = norm(eRot);
if theta_mag < 1e-9
   axisError = [0 0 0];
else
   axisError = (sin(theta_mag/2)/theta_mag) * eRot;
end



error(1) = eWorld(1);
error(2) = eWorld(2);
error(3) = eWorld(3);
error(4) = axisError(1);
error(5) = axisError(2);
error(6) = axisError(3);

end




% error(4) = eVector(1);
% error(5) = eVector(2);
% error(6) = eVector(3);

% function normalizedError = fcn(currentPosition, currentSetPoint)
% 
% normalized = zeros(1,6);
% 
% normalized(1) = -(currentPosition(1) - currentSetPoint(1));
% normalized(2) = -(currentPosition(2) - currentSetPoint(2));
% normalized(3) = -(currentPosition(3) - currentSetPoint(3));
% 
% W2B = [currentPosition(4), currentPosition(5), currentPosition(6), currentPosition(7)];
% setQuat = [currentSetPoint(4), -currentSetPoint(5), -currentSetPoint(6), -currentSetPoint(7)];
% 
% 
% %Talos Heading in Body Frame
% Tbody = [1,0,0,0];
% 
% %Transform from Body 2 World
% B2W = [W2B(1), -W2B(2), -W2B(3), -W2B(4)] / (norm(W2B) ^ 2);
% 
% %Talos Heading in World Frame
% TWorld = quatmultiply(Tbody, B2W);
% 
% %Talos Heading in World Frame Conjugate
% TWorldI = [TWorld(1), -TWorld(2), -TWorld(3), -TWorld(4)];
% 
% %Current Yaw Error
% eQuat = quatmultiply(setQuat, TWorldI);
% 
% % %axis Error
% axisError = [eQuat(2), eQuat(3), eQuat(4)];
% if(eQuat(1) < 0)
%     axisError = -axisError;
% end
% 
% 
% normalized(4) = axisError(1);
% normalized(5) = axisError(2);
% normalized(6) = axisError(3);
% 
% normalizedError = normalized;

== matlab function newController/PID Control2/Enabled Subsystem/MATLAB Function ==
  data: error input; haveGainsChanged input; reset input; currentTime input; prevTime input; prevSum input; sumOfError output
function sumOfError = fcn(error, haveGainsChanged, reset, currentTime, prevTime, prevSum)

dt = 0;
if(prevTime == 0)
    sumOfError = zeros(1,6);
    return
else
    dt = currentTime-prevTime;
end

if(reset || haveGainsChanged)
    sumOfError = zeros(1,6);
    return
end

sumOfError = zeros(1,6);

%check each degree of freedom
for i = 1:6
    sumOfError(i) = (error(i)) * dt + prevSum(i);

    %reset if nan
    if(isnan(error(i)))
        sumOfError(i) = 0;
    end

end

end
